simulink model "Cinematica"  (R2020b)
settings: Solver=VariableStepAuto  StartTime=0.0  StopTime=Smi.general.simulation_time  FixedStep=0.001  MaxStep=0.001  RelTol=1e-3  AbsTol=1e-3  EnableMultiTasking=on
undefined symbols (not defined in the file or in its folder): Smi, X, Y, Z
libraries: sm_lib x99, nesl_utility x24, simulink x1, dspsrcs4 x1, cstblocks x1
(part 1 of 5)
settings Model: Creator=nicop  LastModifiedBy=nicop
settings SolverCC: AutoScaleAbsTol=off
settings DataIOCC: LimitDataPoints=on  MaxDataPoints=10000
settings OptimizationCC: LifeSpan=inf
settings DebuggingCC: ReadBeforeWriteMsg=DisableAll  WriteAfterWriteMsg=DisableAll  WriteAfterReadMsg=DisableAll  MultiTaskDSMMsg=none  AllowSymbolicDim=off  SFUnexpectedBacktrackingDiag=warning  SFNoUnconditionalDefaultTransitionDiag=warning  SFExecutionAtInitializationDiag=none  ArithmeticOperatorsInVariantConditions=warning
settings SFSimCC: SFSimEcho=off  SimUseLocalCustomCode=off  CustomCodeUndefinedFunction=UseInterfaceOnly
settings RTWCC: RTWUseLocalCustomCode=off
settings CodeAppCC: StateflowObjectComments=on
settings GRTTargetCC: TargetLangStandard=C89/C90 (ANSI)
settings ConfigComp: CovMetricSettings=dw  CovSaveCumulativeToWorkspaceVar=on  CovSaveSingleToWorkspaceVar=on  CovExternalEMLEnable=off  CovSFcnEnable=off
settings SimscapeCC: SimscapeLogType=all  SimscapeLogSimulationStatistics=on  SimscapeLogDataHistory=10000

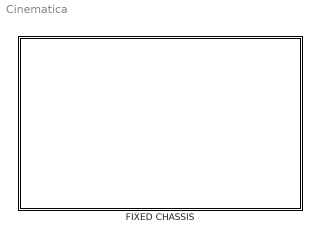
== system Cinematica ==
  FIXED CHASSIS : Subsystem

== system Cinematica/FIXED CHASSIS ==
  ACTUATOR FL : Subsystem
  BODY : Subsystem
      settings: PortSchema="{\"entries\":[{\"content\":{\"sides\":[{\"content\":{\"connectorIds\":[\"LConn1\",\"LConn2\",\"LConn3\",\"LConn4\",\"LConn5\",\"LConn6\",\"LConn7\",\"LConn8\",\"LConn9\"]},\"type\":\"ConnectorPlacement.EquallySpacedRectSide\",\"uuid\":\"4c2bbaf1-fbd8-4943-99e0-470de1938501\"},{\"content\":{\"connectorIds\":[],\"side\":\"RIGHT\"},\"type\":\"ConnectorPlacement.EquallySpacedRectSide\",\"uuid\":\"782ff682-1e99-4a86-9ae1-6b10d64c2634\"},{\"content\":{\"connectorIds\":[\"LConn10\"],\"side\":\"TOP\"},\"type\":\"ConnectorPlacement.EquallySpacedRectSide\",\"uuid\":\"0b3565bb-f882-4cc1-9f6f-7b6d6ef48850\"},{\"content\":{\"connectorIds\":[\"RConn1\"],\"side\":\"BOTTOM\"},\"type\":\"ConnectorPlacement.EquallySpacedRectSide\",\"uuid\":\"2660912b-114d-4160-a2f6-1b97c7cfb4a4\"},{\"content\":{\"connectorIds\":[],\"side\":\"HIDDEN\"},\"type\":\"ConnectorPlacement.EquallySpacedRectSide\",\"uuid\":\"29404510-5925-4bb6-a2d1-6f2b8f5e0381\"}]},\"type\":\"ConnectorPlacement.EquallySpacedConnector\",\"uuid\":\"2c55a6b1-9684-4292-96ca-1ed68c3a6f99\"}],\"packageUris\":[\"http://schema.mathworks.com/mf0/Connector/R2020b\"],\"version\":\"1.0\"}"
  FL SUSPENSION : Subsystem
  WORLD : Subsystem
  connections:
  BODY/LConn7 -- FL SUSPENSION/RConn8
  FL SUSPENSION/RConn5 -- BODY/LConn4
  FL SUSPENSION/RConn4 -- BODY/LConn3
  FL SUSPENSION/LConn2 -- ACTUATOR FL/LConn1
  FL SUSPENSION/RConn7 -- BODY/LConn6
  BODY/LConn9 -- ACTUATOR FL/RConn1
  WORLD/RConn1 -- BODY/RConn1
  FL SUSPENSION/RConn2 -- BODY/LConn1
  BODY/LConn10 -- FL SUSPENSION/RConn1
  BODY/LConn5 -- FL SUSPENSION/RConn6
  FL SUSPENSION/RConn3 -- BODY/LConn2
  FL SUSPENSION/RConn9 -- BODY/LConn8
  ACTUATOR FL/LConn2 -- FL SUSPENSION/LConn1

== system Cinematica/FIXED CHASSIS/ACTUATOR FL ==
  ACTUATOR : Subsystem
  ACTUATOR IN/OUT : Subsystem
  OUTER ACTUATOR : Subsystem
      settings: PortSchema="{\"entries\":[{\"content\":{\"sides\":[{\"content\":{\"connectorIds\":[]},\"type\":\"ConnectorPlacement.EquallySpacedRectSide\",\"uuid\":\"d7e62bfe-6450-4a39-85d3-bed3049c321c\"},{\"content\":{\"connectorIds\":[],\"side\":\"RIGHT\"},\"type\":\"ConnectorPlacement.EquallySpacedRectSide\",\"uuid\":\"3cbc563a-0112-4986-bd57-0cf817b4d4bf\"},{\"content\":{\"connectorIds\":[\"LConn1\"],\"side\":\"TOP\"},\"type\":\"ConnectorPlacement.EquallySpacedRectSide\",\"uuid\":\"eb91a932-1d66-4430-a168-6ec694e02ce0\"},{\"content\":{\"connectorIds\":[\"RConn1\"],\"side\":\"BOTTOM\"},\"type\":\"ConnectorPlacement.EquallySpacedRectSide\",\"uuid\":\"a5a9eb1a-4070-480d-a72b-be2caa4d4ddd\"},{\"content\":{\"connectorIds\":[],\"side\":\"HIDDEN\"},\"type\":\"ConnectorPlacement.EquallySpacedRectSide\",\"uuid\":\"1c33bc41-55ff-4930-aaf8-325eabd2d214\"}]},\"type\":\"ConnectorPlacement.EquallySpacedConnector\",\"uuid\":\"9fea4cfe-800a-4673-925c-b7963aa13243\"}],\"packageUris\":[\"http://schema.mathworks.com/mf0/Connector/R2020b\"],\"version\":\"1.0\"}"
  Full geometry : PMIOPort  Side=Left
  WORLD : PMIOPort  Port=2  Side=Right
  CP : PMIOPort  Port=3  Side=Left
  connections:
  OUTER ACTUATOR/LConn1 -- ACTUATOR IN/OUT/RConn1
  ACTUATOR/LConn2 -- CP/RConn1
  ACTUATOR/LConn1 -- Full geometry/RConn1
  ACTUATOR IN/OUT/LConn1 -- ACTUATOR/RConn1
  WORLD/RConn1 -- OUTER ACTUATOR/RConn1

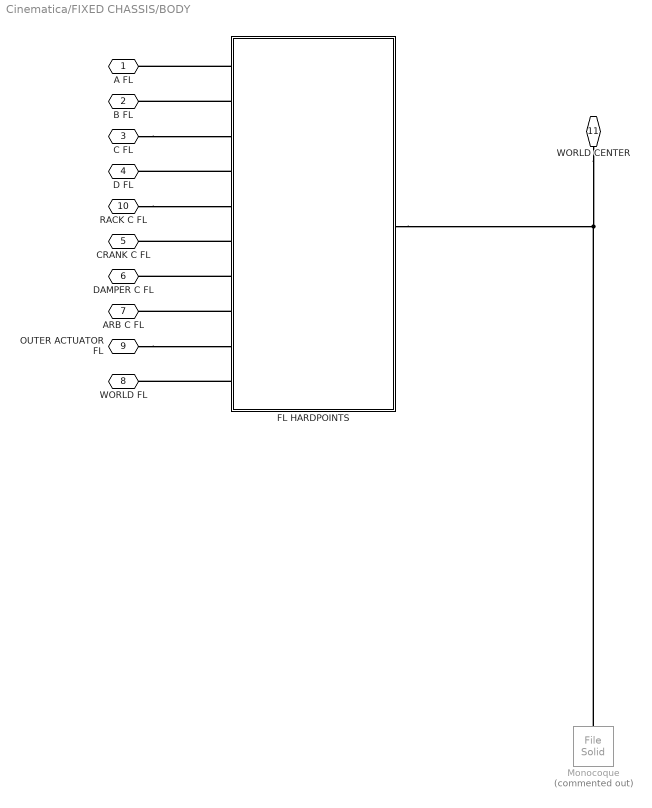
== system Cinematica/FIXED CHASSIS/BODY ==
  FL HARDPOINTS : Subsystem
  Monocoque : sm_lib/Body Elements/File Solid  Commented=on  ExtGeomFileName=Parameters\Monocoque.stp  UnitType=FromFile  ExtGeomFileUnits=m  StepReaderType=HEX  ExportConvexHullGeometry=off  InertiaType=PointMass  Mass=1  MassUnits=kg  CenterOfMass=[0 0 0]  CenterOfMassUnits=m  MomentsOfInertia=[1 1 1]  MomentsOfInertiaUnits=kg*m^2  ProductsOfInertia=[0 0 0]  ProductsOfInertiaUnits=kg*m^2  BasedOnType=DensityFromFile  Density=1000  DensityUnits=kg/m^3  DoExposeReferenceFrame=on  SerializedFrames=<Frames/>  GraphicType=FromGeometry  MarkerShape=Sphere  MarkerSize=10  GraphicVisPropType=SimpleVisualProperties  GraphicDiffuseColor=[1.0 1.0 1.0]  GraphicSpecularColor=[0.5 0.5 0.5 1.0]  GraphicAmbientColor=[0.15 0.15 0.15 1.0]  GraphicEmissiveColor=[0.0 0.0 0.0 1.0]  GraphicShininess=75  GraphicOpacity=0.4
  A FL : PMIOPort  Side=Left
  B FL : PMIOPort  Port=2  Side=Left
  C FL : PMIOPort  Port=3  Side=Left
  D FL : PMIOPort  Port=4  Side=Left
  CRANK C FL : PMIOPort  Port=5  Side=Left
  DAMPER C FL : PMIOPort  Port=6  Side=Left
  ARB C FL : PMIOPort  Port=7  Side=Left
  WORLD FL : PMIOPort  Port=8  Side=Left
  OUTER ACTUATOR FL : PMIOPort  Port=9  Side=Left
  RACK C FL : PMIOPort  Port=10  Side=Left
  WORLD CENTER : PMIOPort  Port=11  Side=Right
  connections:
  FL HARDPOINTS/RConn1 -- Monocoque/RConn1 -- WORLD CENTER/RConn1
  FL HARDPOINTS/LConn10 -- WORLD FL/RConn1
  OUTER ACTUATOR FL/RConn1 -- FL HARDPOINTS/LConn9
  FL HARDPOINTS/LConn8 -- ARB C FL/RConn1
  FL HARDPOINTS/LConn7 -- DAMPER C FL/RConn1
  FL HARDPOINTS/LConn6 -- CRANK C FL/RConn1
  RACK C FL/RConn1 -- FL HARDPOINTS/LConn5
  FL HARDPOINTS/LConn4 -- D FL/RConn1
  C FL/RConn1 -- FL HARDPOINTS/LConn3
  FL HARDPOINTS/LConn2 -- B FL/RConn1
  FL HARDPOINTS/LConn1 -- A FL/RConn1
